simulink model "MATLAB_TEST"  (R2019b)
settings: Solver=FixedStepDiscrete  StartTime=0  StopTime=50  FixedStep=0.0025  RelTol=1e-3
undefined symbols (not defined in the file): BCM_COM_PROC_P20, BCM_COM_PROC_P20_SFW_R2018b, BCM_COM_PROC_P2_5, BCM_COM_PROC_P2_5_SFW_R2018b, BCM_COM_PROC_P5, BCM_COM_PROC_P5_SFW_R2018b, BCMA_ACCU_PT_Conf_Flt, BCMA_ACCU_PT_Unconf_Flt, BCMA_Antiskid_Off_Sanction, BCMA_Avionics_Conf_Flt, BCMA_BCM_CCDL_Conf_Flt, BCMA_BCM_CCDL_Unconf_Flt, BCMA_BCM_DBCU_INHIBITION_Conf_Flt, BCMA_BCM_DBCU_INHIBITION_Unconf_Flt, BCMA_BCP_ALT_Disp_Sw_Conf_Flt, BCMA_BCP_ALT_Disp_Sw_Unconf_Flt, BCMA_BCP_ALT_SW_ON_CMD_Conf_Flt, BCMA_BCP_ALT_SW_ON_CMD_Unconf_Flt, BCMA_BCP_PARK_OFF_SW_CMD_Conf_Flt, BCMA_BCP_PARK_OFF_SW_CMD_Unconf_Flt, BCMA_CF_BSELV_JCL, BCMA_CF_BSELV_JOP, BCMA_CF_BSELV_OC, BCMA_CF_BSELV_SC, BCMA_CF_LH_SV_JCL, BCMA_CF_LH_SV_JOP, BCMA_CF_LH_SV_OC, BCMA_CF_LH_SV_SC, BCMA_CF_PARK_BRK, BCMA_CF_RESIDUAL_PRESS, BCMA_CF_RH_SV_JCL, BCMA_CF_RH_SV_JOP, BCMA_CF_RH_SV_OC, BCMA_CF_RH_SV_SC, BCMA_CF_SELV_JCL, BCMA_CF_SELV_JOP, BCMA_CF_SELV_OC, BCMA_CF_SELV_SC, BCMA_CF_SV_DRIFT, BCMA_DBCU_ALT_MODE_Conf_Flt, BCMA_DBCU_ALT_MODE_Unconf_Flt, BCMA_DBCU_BRK_ORDER_FAIL_Conf_Flt, BCMA_DBCU_BRK_ORDER_FAIL_Unconf_Flt, BCMA_DBCU_Conf_Flt, BCMA_DBCU_DISPATCH_SW_ON_Conf_Flt, BCMA_DBCU_DISPATCH_SW_ON_Unconf_Flt, BCMA_DBCU_FAILED_Conf_Flt, BCMA_DBCU_FAILED_Unconf_Flt, BCMA_DFCS1_Capsule_Validity, BCMA_DFCS1_Label202_Corrupted, BCMA_DFCS1_Label202_Not_Refreshed, BCMA_DFCS1_Label204_Corrupted, BCMA_DFCS1_Label204_Not_Refreshed, BCMA_DFCS1_Label205_Corrupted, BCMA_DFCS1_Label205_Not_Refreshed, BCMA_DFCS1_Label206_Corrupted, BCMA_DFCS1_Label206_Not_Refreshed, BCMA_DFCS1_Label207_Corrupted, BCMA_DFCS1_Label207_Not_Refreshed, BCMA_DFCS3_Capsule_Validity ... (+762)
libraries: simulink x73, lib_MBD_Control x5
(part 8 of 16)

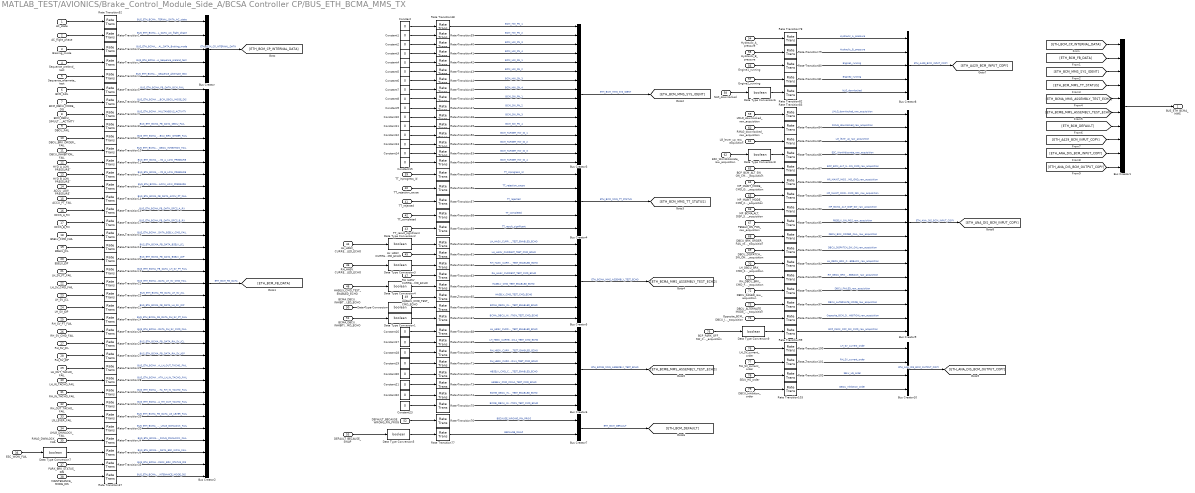
== system MATLAB_TEST/AVIONICS/Brake_Control_Module_Side_A/BCSA Controller CP/BUS_ETH_BCMA_MMS_TX ==
  AC_state : Inport
  AC_flight_phase : Inport  Port=2
  Braking_mode : Inport  Port=3
  Sequence_preland_test : Inport  Port=4
  Sequence_alternate_test : Inport  Port=5
  BCM_FAIL : Inport  Port=6
  BCM_DBCU_MODE_DIS : Inport  Port=7
  BCM_DBCU_SIMULTANEOUS_ACTIVITY : Inport  Port=8
  DBCU_FAIL : Inport  Port=9
  DBCU_BRK_ORDER_FAIL : Inport  Port=10
  DBCU_INHIBITION_FAIL : Inport  Port=11
  HYD_A_LOW_PRESSURE : Inport  Port=12
  HYD_B_LOW_PRESSURE : Inport  Port=13
  ACCU_LOW_PRESSURE : Inport  Port=14
  ACCU_PT_FAIL : Inport  Port=15
  DFCS_A_RX : Inport  Port=16
  DFCS_B_RX : Inport  Port=17
  BSELV_CMD_FAIL : Inport  Port=18
  BSELV_JCL : Inport  Port=19
  BSELV_JOP : Inport  Port=20
  LH_SV_PT_FAIL : Inport  Port=21
  LH_SV_CMD_FAIL : Inport  Port=22
  LH_SV_JCL : Inport  Port=23
  LH_SV_JOP : Inport  Port=24
  RH_SV_PT_FAIL : Inport  Port=25
  RH_SV_CMD_FAIL : Inport  Port=26
  RH_SV_JCL : Inport  Port=27
  RH_SV_JOP : Inport  Port=28
  LH_OUT_TACHO_FAIL : Inport  Port=29
  LH_IN_TACHO_FAIL : Inport  Port=30
  RH_IN_TACHO_FAIL : Inport  Port=31
  RH_OUT_TACHO_FAIL : Inport  Port=32
  LG_LEVER_FAIL : Inport  Port=33
  LMLG_DWNLOCK_FAIL : Inport  Port=34
  RMLG_DWNLOCK_FAIL : Inport  Port=35
  ESC_WOW_FAIL : Inport  Port=36
  PARK_BRK_STATUS_DIS : Inport  Port=37
  MAINTENANCE_MODE_DIS : Inport  Port=38
  TT_inprogress_id : Inport  Port=39
  TT_rejection_cause : Inport  Port=40
  TT_rejected : Inport  Port=41
  TT_completed : Inport  Port=42
  TT_result_significant : Inport  Port=43
  LH_HASV_CURRENT_TEST_ENABLED_ECHO : Inport  Port=44
  LH_HASV_CURRENT_TEST_CMD_ECHO : Inport  Port=45
  RH_HASV_CURRENT_TEST_ENABLED_ECHO : Inport  Port=46
  RH_HASV_CURRENT_TEST_CMD_ECHO : Inport  Port=47
  HASELV_CMD_TEST_ENABLED_ECHO : Inport  Port=48
  HASELV_CMD_TEST_CMD_ECHO : Inport  Port=49
  BCMA_DBCU_INHIBITION_TEST_ENABLED_ECHO : Inport  Port=50
  BCMA_DBCU_INHIBITION_TEST_CMD_ECHO : Inport  Port=51
  DEFAULT_BECAUSE_WRONG_PIN_PROG : Inport  Port=52
  DEFAULT_BECAUSE_SWAP : Inport  Port=53
  Hydraulic_A_pressure : Inport  Port=54
  Hydraulic_B_pressure : Inport  Port=55
  Engine1_running : Inport  Port=56
  Engine2_running : Inport  Port=57
  NLG_downlocked : Inport  Port=58
  LMLG_downlocked_raw_acquisition : Inport  Port=59
  RMLG_downlocked_raw_acquisition : Inport  Port=60
  LG_lever_up_raw_acquisition : Inport  Port=61
  ESC_WonWdiscrete_raw_acquisition : Inport  Port=62
  BCP_BCM_ALT_SW_ON_CMD_raw_acquisition : Inport  Port=63
  MP_MAINT_MODE_CMD_GND_raw_acquisition : Inport  Port=64
  MP_MAINT_MODE_CMD_28V_raw_acquisition : Inport  Port=65
  MP_BCMA_ALT_DISP_SW_raw_acquisition : Inport  Port=66
  PBSELV_ON_POS_raw_acquisition : Inport  Port=67
  DBCU_BRK_ORDER_FAIL_raw_acquisition : Inport  Port=68
  DBCU_DISPATCH_SW_ON_raw_acquisition : Inport  Port=69
  LH_DBCU_BRK_CMD_FEEDBACK_raw_acquisition : Inport  Port=70
  RH_DBCU_BRK_CMD_FEEDBACK_raw_acquisition : Inport  Port=71
  DBCU_FAILED_raw_acquisition : Inport  Port=72
  DBCU_ALTERNATE_MODE_raw_acquisition : Inport  Port=73
  Opposite_BCM_DBCU_INHIBITION_raw_acquisition : Inport  Port=74
  BCP_PARK_OFF_SW_CMD_raw_acquisition : Inport  Port=75
  LH_SV_current_order : Inport  Port=76
  RH_SV_current_order : Inport  Port=77
  SELV_HS_order : Inport  Port=78
  DBCU_Inhibition_order : Inport  Port=79
  Bus Creator : BusCreator  Inputs=5  OutDataTypeStr=Bus: BUS_ETH_BCM_CP_INTERNAL_DATA  NonVirtualBus=on
  Bus Creator1 : BusCreator  Inputs=10  OutDataTypeStr=Bus: BUS_ETH_BCMB_MMS  NonVirtualBus=on
      settings: InheritFromInputs=off
  Bus Creator10 : BusCreator  Inputs=4  OutDataTypeStr=Bus: BUS_ETH_ANA_DIS_BCM_OUTPUT_COPY  NonVirtualBus=on
      settings: InheritFromInputs=off
  Bus Creator2 : BusCreator  Inputs=33  OutDataTypeStr=Bus: BUS_ETH_BCM_FB_DATA  NonVirtualBus=on
      settings: InheritFromInputs=off
  Bus Creator3 : BusCreator  Inputs=16  OutDataTypeStr=Bus: BUS_ETH_BCM_MMS_SYS_IDENT  NonVirtualBus=on
      settings: InheritFromInputs=off
  Bus Creator4 : BusCreator  Inputs=5  OutDataTypeStr=Bus: BUS_ETH_BCM_MMS_TT_STATUS  NonVirtualBus=on
      settings: InheritFromInputs=off
  Bus Creator5 : BusCreator  Inputs=8  OutDataTypeStr=Bus: BUS_ETH_BCMA_MMS_ASSEMBLY_TEST_ECHO  NonVirtualBus=on
      settings: InheritFromInputs=off
  Bus Creator6 : BusCreator  Inputs=8  OutDataTypeStr=Bus: BUS_ETH_BCMB_MMS_ASSEMBLY_TEST_ECHO  NonVirtualBus=on
      settings: InheritFromInputs=off
  Bus Creator7 : BusCreator  Inputs=2  OutDataTypeStr=Bus: BUS_ETH_BCM_DEFAULT  NonVirtualBus=on
      settings: InheritFromInputs=off
  Bus Creator8 : BusCreator  Inputs=5  OutDataTypeStr=Bus: BUS_ETH_A429_BCM_INPUT_COPY  NonVirtualBus=on
      settings: InheritFromInputs=off
  Bus Creator9 : BusCreator  Inputs=17  OutDataTypeStr=Bus: BUS_ETH_ANA_DIS_BCM_INPUT_COPY  NonVirtualBus=on
      settings: InheritFromInputs=off
  Constant{,1..16,18,20,22..23} (21 alike) : Constant  Value=0  OutDataTypeStr=boolean
  Constant17 : Constant  Value=0  OutDataTypeStr=int32
  Constant19 : Constant  Value=0  OutDataTypeStr=int32
  Constant21 : Constant  Value=0  OutDataTypeStr=int32
  Data Type Conversion{,1..9} (10 alike) : DataTypeConversion  OutDataTypeStr=boolean
  Rate Transition{1..103} (103 alike) : RateTransition  Deterministic=off  OutPortSampleTime=1/10
      settings: AttributesFormatString=OutPortSampleTime %<OutPortSampleTime>
  BUS_ETH_BCMA_MMS : Outport  VectorParamsAs1DForOutWhenUnconnected=off
  wires:
  Bus Creator/1 -> [ETH_BCM_CP_INTERNAL_DATA]  "ETH_BCM_CP_INTERNAL_DATA"
  AC_flight_phase/1 -> Rate Transition1/1
  Braking_mode/1 -> Rate Transition2/1
  Sequence_preland_test/1 -> Rate Transition3/1
  Sequence_alternate_test/1 -> Rate Transition4/1
  Bus Creator1/1 -> BUS_ETH_BCMA_MMS/1
  Bus Creator2/1 -> [ETH_BCM_FB_DATA]  "ETH_BCM_FB_DATA"
  BCM_FAIL/1 -> Rate Transition5/1
  BCM_DBCU_MODE_DIS/1 -> Rate Transition6/1
  BCM_DBCU_SIMULTANEOUS_ACTIVITY/1 -> Rate Transition7/1
  DBCU_FAIL/1 -> Rate Transition8/1
  DBCU_BRK_ORDER_FAIL/1 -> Rate Transition9/1
  DBCU_INHIBITION_FAIL/1 -> Rate Transition10/1
  HYD_A_LOW_PRESSURE/1 -> Rate Transition11/1
  HYD_B_LOW_PRESSURE/1 -> Rate Transition12/1
  ACCU_LOW_PRESSURE/1 -> Rate Transition13/1
  ACCU_PT_FAIL/1 -> Rate Transition14/1
  DFCS_A_RX/1 -> Rate Transition15/1
  DFCS_B_RX/1 -> Rate Transition17/1
  BSELV_CMD_FAIL/1 -> Rate Transition16/1
  BSELV_JCL/1 -> Rate Transition18/1
  BSELV_JOP/1 -> Rate Transition20/1
  LH_SV_PT_FAIL/1 -> Rate Transition19/1
  LH_SV_CMD_FAIL/1 -> Rate Transition21/1
  LH_SV_JCL/1 -> Rate Transition23/1
  LH_SV_JOP/1 -> Rate Transition22/1
  RH_SV_PT_FAIL/1 -> Rate Transition24/1
  RH_SV_CMD_FAIL/1 -> Rate Transition26/1
  RH_SV_JCL/1 -> Rate Transition25/1
  RH_SV_JOP/1 -> Rate Transition27/1
  LH_OUT_TACHO_FAIL/1 -> Rate Transition29/1
  LH_IN_TACHO_FAIL/1 -> Rate Transition28/1
  RH_IN_TACHO_FAIL/1 -> Rate Transition30/1
  RH_OUT_TACHO_FAIL/1 -> Rate Transition31/1
  LG_LEVER_FAIL/1 -> Rate Transition33/1
  LMLG_DWNLOCK_FAIL/1 -> Rate Transition32/1
  RMLG_DWNLOCK_FAIL/1 -> Rate Transition34/1
  ESC_WOW_FAIL/1 -> Data Type Conversion7/1
  PARK_BRK_STATUS_DIS/1 -> Rate Transition35/1
  MAINTENANCE_MODE_DIS/1 -> Rate Transition37/1
  Constant/1 -> Rate Transition38/1
  Constant1/1 -> Rate Transition39/1
  Constant2/1 -> Rate Transition40/1
  Constant3/1 -> Rate Transition41/1
  Constant4/1 -> Rate Transition42/1
  Constant5/1 -> Rate Transition43/1
  Constant6/1 -> Rate Transition44/1
  Constant7/1 -> Rate Transition45/1
  Constant8/1 -> Rate Transition46/1
  Constant9/1 -> Rate Transition47/1
  Constant10/1 -> Rate Transition48/1
  Constant11/1 -> Rate Transition49/1
  Constant12/1 -> Rate Transition50/1
  Constant13/1 -> Rate Transition51/1
  Constant14/1 -> Rate Transition53/1
  Constant15/1 -> Rate Transition54/1
  [ETH_BCM_CP_INTERNAL_DATA] -> Bus Creator1/1
  [ETH_BCM_FB_DATA] -> Bus Creator1/2
  Bus Creator3/1 -> [ETH_BCM_MMS_SYS_IDENT]  "ETH_BCM_MMS_SYS_IDENT"
  [ETH_BCM_MMS_SYS_IDENT] -> Bus Creator1/3
  TT_result_significant/1 -> Rate Transition59/1
  TT_completed/1 -> Rate Transition58/1
  TT_rejected/1 -> Rate Transition57/1
  TT_rejection_cause/1 -> Rate Transition56/1
  TT_inprogress_id/1 -> Rate Transition55/1
  Bus Creator4/1 -> [ETH_BCM_MMS_TT_STATUS]  "ETH_BCM_MMS_TT_STATUS"
  [ETH_BCM_MMS_TT_STATUS] -> Bus Creator1/4
  Bus Creator5/1 -> [ETH_BCMA_MMS_ASSEMBLY_TEST_ECHO]  "ETH_BCMA_MMS_ASSEMBLY_TEST_ECHO"
  [ETH_BCMA_MMS_ASSEMBLY_TEST_ECHO] -> Bus Creator1/5
  LH_HASV_CURRENT_TEST_ENABLED_ECHO/1 -> Data Type Conversion2/1
  LH_HASV_CURRENT_TEST_CMD_ECHO/1 -> Rate Transition61/1
  RH_HASV_CURRENT_TEST_ENABLED_ECHO/1 -> Data Type Conversion3/1
  RH_HASV_CURRENT_TEST_CMD_ECHO/1 -> Rate Transition63/1
  HASELV_CMD_TEST_ENABLED_ECHO/1 -> Data Type Conversion4/1
  HASELV_CMD_TEST_CMD_ECHO/1 -> Rate Transition65/1
  BCMA_DBCU_INHIBITION_TEST_ENABLED_ECHO/1 -> Data Type Conversion/1
  BCMA_DBCU_INHIBITION_TEST_CMD_ECHO/1 -> Data Type Conversion1/1
  Constant23/1 -> Rate Transition75/1
  Constant22/1 -> Rate Transition74/1
  Constant21/1 -> Rate Transition73/1
  Constant20/1 -> Rate Transition72/1
  Constant19/1 -> Rate Transition71/1
  Constant18/1 -> Rate Transition70/1
  Constant17/1 -> Rate Transition69/1
  Constant16/1 -> Rate Transition68/1
  Bus Creator6/1 -> [ETH_BCMB_MMS_ASSEMBLY_TEST_ECHO]  "ETH_BCMB_MMS_ASSEMBLY_TEST_ECHO"
  [ETH_BCMB_MMS_ASSEMBLY_TEST_ECHO] -> Bus Creator1/6
  DEFAULT_BECAUSE_SWAP/1 -> Data Type Conversion5/1
  DEFAULT_BECAUSE_WRONG_PIN_PROG/1 -> Rate Transition76/1
  Bus Creator7/1 -> [ETH_BCM_DEFAULT]  "ETH_BCM_DEFAULT"
  [ETH_BCM_DEFAULT] -> Bus Creator1/7
  Rate Transition52/1 -> Bus Creator/1  "BUS_ETH_BCMA_CP_INTERNAL_DATA_AC_state"
  Rate Transition1/1 -> Bus Creator/2  "BUS_ETH_BCMA_CP_INTERNAL_DATA_AC_flight_phase"
  Rate Transition2/1 -> Bus Creator/3  "BUS_ETH_BCMA_CP_INTERNAL_DATA_Braking_mode"
  Rate Transition3/1 -> Bus Creator/4  "BUS_ETH_BCMA_CP_INTERNAL_DATA_Sequence_preland_test"
  Rate Transition4/1 -> Bus Creator/5  "BUS_ETH_BCMA_CP_INTERNAL_DATA_Sequence_alternate_test"
  Rate Transition5/1 -> Bus Creator2/1  "BUS_ETH_BCMA_FB_DATA_BCM_FAIL"
  Rate Transition6/1 -> Bus Creator2/2  "BUS_ETH_BCMA_FB_DATA_BCM_DBCU_MODE_DIS"
  Rate Transition7/1 -> Bus Creator2/3  "BUS_ETH_BCMA_FB_DATA_BCM_DBCU_SIMULTANEOUS_ACTIVITY"
  Rate Transition8/1 -> Bus Creator2/4  "BUS_ETH_BCMA_FB_DATA_DBCU_FAIL"
  Rate Transition9/1 -> Bus Creator2/5  "BUS_ETH_BCMA_FB_DATA_DBCU_BRK_ORDER_FAIL"
  Rate Transition10/1 -> Bus Creator2/6  "BUS_ETH_BCMA_FB_DATA_DBCU_INHIBITION_FAIL"
  Rate Transition11/1 -> Bus Creator2/7  "BUS_ETH_BCMA_FB_DATA_HYD_A_LOW_PRESSURE"
  Rate Transition12/1 -> Bus Creator2/8  "BUS_ETH_BCMA_FB_DATA_HYD_B_LOW_PRESSURE"
  Rate Transition13/1 -> Bus Creator2/9  "BUS_ETH_BCMA_FB_DATA_ACCU_LOW_PRESSURE"
  Rate Transition14/1 -> Bus Creator2/10  "BUS_ETH_BCMA_FB_DATA_ACCU_PT_FAIL"
  Rate Transition16/1 -> Bus Creator2/13  "BUS_ETH_BCMA_FB_DATA_BSELV_CMD_FAIL"
  Rate Transition15/1 -> Bus Creator2/11  "BUS_ETH_BCMA_FB_DATA_DFCS_A_RX"
  Rate Transition17/1 -> Bus Creator2/12  "BUS_ETH_BCMA_FB_DATA_DFCS_B_RX"
  Rate Transition18/1 -> Bus Creator2/14  "BUS_ETH_BCMA_FB_DATA_BSELV_JCL"
  Rate Transition20/1 -> Bus Creator2/15  "BUS_ETH_BCMA_FB_DATA_BSELV_JOP"
  Rate Transition19/1 -> Bus Creator2/16  "BUS_ETH_BCMA_FB_DATA_LH_SV_PT_FAIL"
  Rate Transition23/1 -> Bus Creator2/18  "BUS_ETH_BCMA_FB_DATA_LH_SV_JCL"
  Rate Transition22/1 -> Bus Creator2/19  "BUS_ETH_BCMA_FB_DATA_LH_SV_JOP"
  Rate Transition21/1 -> Bus Creator2/17  "BUS_ETH_BCMA_FB_DATA_LH_SV_CMD_FAIL"
  Rate Transition26/1 -> Bus Creator2/21  "BUS_ETH_BCMA_FB_DATA_RH_SV_CMD_FAIL"
  Rate Transition25/1 -> Bus Creator2/22  "BUS_ETH_BCMA_FB_DATA_RH_SV_JCL"
  Rate Transition24/1 -> Bus Creator2/20  "BUS_ETH_BCMA_FB_DATA_RH_SV_PT_FAIL"
  Rate Transition29/1 -> Bus Creator2/24  "BUS_ETH_BCMA_FB_DATA_LH_OUT_TACHO_FAIL"
  Rate Transition27/1 -> Bus Creator2/23  "BUS_ETH_BCMA_FB_DATA_RH_SV_JOP"
  Rate Transition28/1 -> Bus Creator2/25  "BUS_ETH_BCMA_FB_DATA_LH_IN_TACHO_FAIL"
  Rate Transition36/1 -> Bus Creator2/31  "BUS_ETH_BCMA_FB_DATA_ESC_WOW_FAIL"
  Rate Transition35/1 -> Bus Creator2/32  "BUS_ETH_BCMA_FB_DATA_PARK_BRK_STATUS_DIS"
  Rate Transition34/1 -> Bus Creator2/30  "BUS_ETH_BCMA_FB_DATA_RMLG_DWNLOCK_FAIL"
  Rate Transition31/1 -> Bus Creator2/27  "BUS_ETH_BCMA_FB_DATA_RH_OUT_TACHO_FAIL"
  Rate Transition32/1 -> Bus Creator2/29  "BUS_ETH_BCMA_FB_DATA_LMLG_DWNLOCK_FAIL"
  Rate Transition30/1 -> Bus Creator2/26  "BUS_ETH_BCMA_FB_DATA_RH_IN_TACHO_FAIL"
  Rate Transition33/1 -> Bus Creator2/28  "BUS_ETH_BCMA_FB_DATA_LG_LEVER_FAIL"
  Rate Transition37/1 -> Bus Creator2/33  "BUS_ETH_BCMA_FB_DATA_MAINTENANCE_MODE_DIS"
  AC_state/1 -> Rate Transition52/1
  Rate Transition38/1 -> Bus Creator3/1  "BCM_HW_PN_1"
  Rate Transition39/1 -> Bus Creator3/2  "BCM_HW_PN_2"
  Rate Transition40/1 -> Bus Creator3/3  "BCM_HW_PN_3"
  Rate Transition41/1 -> Bus Creator3/4  "BCM_HW_PN_4"
  Rate Transition42/1 -> Bus Creator3/5  "BCM_HW_SN_1"
  Rate Transition43/1 -> Bus Creator3/6  "BCM_HW_SN_2"
  Rate Transition44/1 -> Bus Creator3/7  "BCM_HW_SN_3"
  Rate Transition45/1 -> Bus Creator3/8  "BCM_HW_SN_4"
  Rate Transition46/1 -> Bus Creator3/9  "BCM_SW_PN_1"
  Rate Transition47/1 -> Bus Creator3/10  "BCM_SW_PN_2"
  Rate Transition50/1 -> Bus Creator3/13  "BCM_TARGET_HW_ID_1"
  Rate Transition49/1 -> Bus Creator3/12  "BCM_SW_PN_4"
  Rate Transition48/1 -> Bus Creator3/11  "BCM_SW_PN_3"
  Rate Transition51/1 -> Bus Creator3/14  "BCM_TARGET_HW_ID_2"
  Rate Transition53/1 -> Bus Creator3/15  "BCM_TARGET_HW_ID_3"
  Rate Transition54/1 -> Bus Creator3/16  "BCM_TARGET_HW_ID_4"
  Rate Transition55/1 -> Bus Creator4/1  "TT_inprogress_id"
  Rate Transition56/1 -> Bus Creator4/2  "TT_rejection_cause"
  Rate Transition57/1 -> Bus Creator4/3  "TT_rejected"
  Rate Transition58/1 -> Bus Creator4/4  "TT_completed"
  Rate Transition59/1 -> Bus Creator4/5  "TT_result_significant"
  Rate Transition60/1 -> Bus Creator5/1  "LH_HASV_CURRENT_TEST_ENABLED_ECHO"
  Rate Transition61/1 -> Bus Creator5/2  "LH_HASV_CURRENT_TEST_CMD_ECHO"
  Rate Transition62/1 -> Bus Creator5/3  "RH_HASV_CURRENT_TEST_ENABLED_ECHO"
  Rate Transition63/1 -> Bus Creator5/4  "RH_HASV_CURRENT_TEST_CMD_ECHO"
  Rate Transition64/1 -> Bus Creator5/5  "HASELV_CMD_TEST_ENABLED_ECHO"
  Rate Transition65/1 -> Bus Creator5/6  "HASELV_CMD_TEST_CMD_ECHO"
  Rate Transition66/1 -> Bus Creator5/7  "BCMA_DBCU_INHIBITION_TEST_ENABLED_ECHO"
  Rate Transition67/1 -> Bus Creator5/8  "BCMA_DBCU_INHIBITION_TEST_CMD_ECHO"
  Rate Transition68/1 -> Bus Creator6/1  "LH_HBSV_CURRENT_COIL1_TEST_ENABLED_ECHO"
  Rate Transition69/1 -> Bus Creator6/2  "LH_HBSV_CURRENT_COIL1_TEST_CMD_ECHO"
  Rate Transition70/1 -> Bus Creator6/3  "RH_HBSV_CURRENT_COIL1_TEST_ENABLED_ECHO"
  Rate Transition71/1 -> Bus Creator6/4  "RH_HBSV_CURRENT_COIL1_TEST_CMD_ECHO"
  Rate Transition72/1 -> Bus Creator6/5  "HBSELV_CMD_COIL1_TEST_ENABLED_ECHO"
  Rate Transition73/1 -> Bus Creator6/6  "HBSELV_CMD_COIL1_TEST_CMD_ECHO"
  Rate Transition74/1 -> Bus Creator6/7  "BCMB_DBCU_INHIBITION_TEST_ENABLED_ECHO"
  Rate Transition75/1 -> Bus Creator6/8  "BCMB_DBCU_INHIBITION_TEST_CMD_ECHO"
  Rate Transition76/1 -> Bus Creator7/1  "BECAUSE_WRONG_PIN_PROG"
  Rate Transition77/1 -> Bus Creator7/2  "BECAUSE_SWAP"
  Hydraulic_A_pressure/1 -> Rate Transition78/1
  Hydraulic_B_pressure/1 -> Rate Transition79/1
  Engine1_running/1 -> Rate Transition80/1
  Engine2_running/1 -> Rate Transition81/1
  NLG_downlocked/1 -> Data Type Conversion6/1
  Rate Transition78/1 -> Bus Creator8/1  "Hydraulic_A_pressure"
  Rate Transition79/1 -> Bus Creator8/2  "Hydraulic_B_pressure"
  Rate Transition80/1 -> Bus Creator8/3  "Engine1_running"
  Rate Transition81/1 -> Bus Creator8/4  "Engine2_running"
  Rate Transition82/1 -> Bus Creator8/5  "NLG_downlocked"
  Bus Creator8/1 -> [ETH_A429_BCM_INPUT_COPY]  "ETH_A429_BCM_INPUT_COPY"
  [ETH_A429_BCM_INPUT_COPY] -> Bus Creator1/8
  Rate Transition83/1 -> Bus Creator9/1  "LMLG_downlocked_raw_acquisition"
  Rate Transition84/1 -> Bus Creator9/2  "RMLG_downlocked_raw_acquisition"
  Rate Transition86/1 -> Bus Creator9/4  "ESC_WonWdiscrete_raw_acquisition"
  Rate Transition85/1 -> Bus Creator9/3  "LG_lever_up_raw_acquisition"
  Rate Transition87/1 -> Bus Creator9/5  "BCP_BCM_ALT_SW_ON_CMD_raw_acquisition"
  Rate Transition88/1 -> Bus Creator9/6  "MP_MAINT_MODE_CMD_GND_raw_acquisition"
  Rate Transition89/1 -> Bus Creator9/7  "MP_MAINT_MODE_CMD_28V_raw_acquisition"
  Rate Transition90/1 -> Bus Creator9/8  "MP_BCMA_ALT_DISP_SW_raw_acquisition"
  Rate Transition91/1 -> Bus Creator9/9  "PBSELV_ON_POS_raw_acquisition"
  Rate Transition92/1 -> Bus Creator9/10  "DBCU_BRK_ORDER_FAIL_raw_acquisition"
  Rate Transition93/1 -> Bus Creator9/11  "DBCU_DISPATCH_SW_ON_raw_acquisition"
  Rate Transition94/1 -> Bus Creator9/12  "LH_DBCU_BRK_CMD_FEEDBACK_raw_acquisition"
  Rate Transition95/1 -> Bus Creator9/13  "RH_DBCU_BRK_CMD_FEEDBACK_raw_acquisition"
  Rate Transition96/1 -> Bus Creator9/14  "DBCU_FAILED_raw_acquisition"
  Rate Transition97/1 -> Bus Creator9/15  "DBCU_ALTERNATE_MODE_raw_acquisition"
  Rate Transition98/1 -> Bus Creator9/16  "Opposite_BCM_DBCU_INHIBITION_raw_acquisition"
  Rate Transition99/1 -> Bus Creator9/17  "BCP_PARK_OFF_SW_CMD_raw_acquisition"
  LMLG_downlocked_raw_acquisition/1 -> Rate Transition83/1
  RMLG_downlocked_raw_acquisition/1 -> Rate Transition84/1
  LG_lever_up_raw_acquisition/1 -> Rate Transition85/1
  ESC_WonWdiscrete_raw_acquisition/1 -> Data Type Conversion8/1
  MP_MAINT_MODE_CMD_GND_raw_acquisition/1 -> Rate Transition88/1
  BCP_BCM_ALT_SW_ON_CMD_raw_acquisition/1 -> Rate Transition87/1
  MP_MAINT_MODE_CMD_28V_raw_acquisition/1 -> Rate Transition89/1
  MP_BCMA_ALT_DISP_SW_raw_acquisition/1 -> Rate Transition90/1
  PBSELV_ON_POS_raw_acquisition/1 -> Rate Transition91/1
  DBCU_BRK_ORDER_FAIL_raw_acquisition/1 -> Rate Transition92/1
  DBCU_DISPATCH_SW_ON_raw_acquisition/1 -> Rate Transition93/1
  LH_DBCU_BRK_CMD_FEEDBACK_raw_acquisition/1 -> Rate Transition94/1
  RH_DBCU_BRK_CMD_FEEDBACK_raw_acquisition/1 -> Rate Transition95/1
  DBCU_FAILED_raw_acquisition/1 -> Rate Transition96/1
  DBCU_ALTERNATE_MODE_raw_acquisition/1 -> Rate Transition97/1
  Opposite_BCM_DBCU_INHIBITION_raw_acquisition/1 -> Rate Transition98/1
  BCP_PARK_OFF_SW_CMD_raw_acquisition/1 -> Data Type Conversion9/1
  Bus Creator9/1 -> [ETH_ANA_DIS_BCM_INPUT_COPY]  "ETH_ANA_DIS_BCM_INPUT_COPY"
  [ETH_ANA_DIS_BCM_INPUT_COPY] -> Bus Creator1/9
  Bus Creator10/1 -> [ETH_ANA_DIS_BCM_OUTPUT_COPY]  "ETH_ANA_DIS_BCM_OUTPUT_COPY"
  [ETH_ANA_DIS_BCM_OUTPUT_COPY] -> Bus Creator1/10
  Rate Transition100/1 -> Bus Creator10/1  "LH_SV_current_order"
  LH_SV_current_order/1 -> Rate Transition100/1
  RH_SV_current_order/1 -> Rate Transition101/1
  SELV_HS_order/1 -> Rate Transition102/1
  DBCU_Inhibition_order/1 -> Rate Transition103/1
  Rate Transition101/1 -> Bus Creator10/2  "RH_SV_current_order"
  Rate Transition102/1 -> Bus Creator10/3  "SELV_HS_order"
  Rate Transition103/1 -> Bus Creator10/4  "DBCU_Inhibition_order"
  Data Type Conversion/1 -> Rate Transition66/1
  Data Type Conversion1/1 -> Rate Transition67/1
  Data Type Conversion2/1 -> Rate Transition60/1
  Data Type Conversion3/1 -> Rate Transition62/1
  Data Type Conversion4/1 -> Rate Transition64/1
  Data Type Conversion5/1 -> Rate Transition77/1
  Data Type Conversion6/1 -> Rate Transition82/1
  Data Type Conversion7/1 -> Rate Transition36/1
  Data Type Conversion8/1 -> Rate Transition86/1
  Data Type Conversion9/1 -> Rate Transition99/1

== system MATLAB_TEST/AVIONICS/Brake_Control_Module_Side_A/BCSA Controller CP/COM_CAN_MON_TX ==
  V_BCM_COM_Braking_Norm_FT_Seq : Inport  SampleTime=0.005
  V_BCM_COM_Braking_Alt_FT_Seq : Inport  Port=2  SampleTime=0.005
  V_BCM_COM_BCM_Validity : Inport  Port=3  SampleTime=0.005
  V_BCM_COM_Norm_Brkg_Availability : Inport  Port=4  SampleTime=0.005
  Bus Creator : BusCreator  Inputs=4
  COM_CAN_MON : Outport  OutputWhenDisabled=reset  InitialOutput=0  VectorParamsAs1DForOutWhenUnconnected=off
      settings: AttributesFormatString=|
      | OutputWhenDisabled %<OutputWhenDisabled>
      | InitialOutput %<InitialOutput>
  wires:
  V_BCM_COM_Braking_Norm_FT_Seq/1 -> Bus Creator/1
  V_BCM_COM_Braking_Alt_FT_Seq/1 -> Bus Creator/2
  V_BCM_COM_BCM_Validity/1 -> Bus Creator/3
  V_BCM_COM_Norm_Brkg_Availability/1 -> Bus Creator/4
  Bus Creator/1 -> COM_CAN_MON/1

== system MATLAB_TEST/AVIONICS/Brake_Control_Module_Side_A/BCSA Controller CP/DBCU Inhibition Failure Mode ==
  DBCU_Inhib_Order : Inport
  Erroneous_DBCU_Activation_Off : Inport  Port=2  SampleTime=0.02
  Erroneous_DBCU_Activation_On : Inport  Port=3  SampleTime=0.02
  AIG3 : lib_MBD_Control/Logics/Signal Routing/AIG3  Tag=AIG4
      settings: SourceProductName=MBD
  Constant1 : Constant  Value=0  OutDataTypeStr=boolean  SampleTime=0.02
  Constant58 : Constant  OutDataTypeStr=boolean  SampleTime=0.02
  DBCU_INHIBITION : Outport  VectorParamsAs1DForOutWhenUnconnected=off
  wires:
  DBCU_Inhib_Order/1 -> AIG3/5
  Erroneous_DBCU_Activation_Off/1 -> AIG3/1
  Erroneous_DBCU_Activation_On/1 -> AIG3/2
  AIG3/1 -> DBCU_INHIBITION/1
  Constant58/1 -> AIG3/3
  Constant1/1 -> AIG3/4

== system MATLAB_TEST/AVIONICS/Brake_Control_Module_Side_A/BCSA Controller CP/DFCS1_Label204_Validity ==
  Capsule_Validity : Inport
  Label204_Not_Refreshed : Inport  Port=2
  Label204_Corrupted : Inport  Port=3
  Label204_SSM : Inport  Port=4
  Compare To Constant : simulink/Logic and Bit Operations/Compare To Constant  relop=~=  const=0  OutDataTypeStr=boolean
  Compare To Zero : simulink/Logic and Bit Operations/Compare To Zero  relop===  OutDataTypeStr=boolean
  Logical Operator : Logic  Operator=OR  Inputs=4  AllPortsSameDT=off  OutDataTypeStr=boolean
  Logical Operator5 : Logic  Operator=NOT  AllPortsSameDT=off  OutDataTypeStr=boolean
  Mux{16,18,20,22} (4 alike) : Mux  Inputs=3
  WOWs_Val_Val : Outport  VectorParamsAs1DForOutWhenUnconnected=off
  LMLG_WOWs_Val : Outport  Port=2  VectorParamsAs1DForOutWhenUnconnected=off
  RMLG_WOWs_Val : Outport  Port=3  VectorParamsAs1DForOutWhenUnconnected=off
  NLG_WOWs_Val : Outport  Port=4  VectorParamsAs1DForOutWhenUnconnected=off
  TLA_Above_Idle_Val : Outport  Port=5  VectorParamsAs1DForOutWhenUnconnected=off
  DCL_Inhibition_Val : Outport  Port=6  VectorParamsAs1DForOutWhenUnconnected=off
  ALT_Mode_1_Val : Outport  Port=7  VectorParamsAs1DForOutWhenUnconnected=off
  ALT_Mode_2_Val : Outport  Port=8  VectorParamsAs1DForOutWhenUnconnected=off
  wires:
  Logical Operator/1 -> Logical Operator5/1
  Mux16/1 -> WOWs_Val_Val/1
  Mux18/1 -> LMLG_WOWs_Val/1
  Mux20/1 -> RMLG_WOWs_Val/1
  Mux22/1 -> NLG_WOWs_Val/1
  Capsule_Validity/1 -> Compare To Zero/1
  Compare To Zero/1 -> Logical Operator/1
  Label204_Not_Refreshed/1 -> Logical Operator/2
  Label204_SSM/1 -> Compare To Constant/1
  Label204_Corrupted/1 -> Logical Operator/3
  Logical Operator5/1 -> ALT_Mode_2_Val/1, ALT_Mode_1_Val/1, DCL_Inhibition_Val/1, TLA_Above_Idle_Val/1, Mux22/3, Mux22/2, Mux22/1, Mux20/3, Mux20/2, Mux20/1, Mux18/3, Mux18/2, Mux18/1, Mux16/3, Mux16/2, Mux16/1
  Compare To Constant/1 -> Logical Operator/4

== system MATLAB_TEST/AVIONICS/Brake_Control_Module_Side_A/BCSA Controller CP/DFCS1_Label205_Validity ==
  Capsule_Validity : Inport
  Label205_Not_Refreshed : Inport  Port=2
  Label205_Corrupted : Inport  Port=3
  Label205_SSM : Inport  Port=4
  DFCSA_Long_Accel : Inport  Port=5
  Compare To Constant : simulink/Logic and Bit Operations/Compare To Constant  relop=~=  const=3.0  OutDataTypeStr=boolean
  Compare To Constant3 : simulink/Logic and Bit Operations/Compare To Constant  relop=<  const=-4  OutDataTypeStr=boolean
  Compare To Constant4 : simulink/Logic and Bit Operations/Compare To Constant  relop=>  const=4  OutDataTypeStr=boolean
  Compare To Zero : simulink/Logic and Bit Operations/Compare To Zero  relop===  OutDataTypeStr=boolean
  Logical Operator1 : Logic  Operator=OR  Inputs=6  AllPortsSameDT=off  OutDataTypeStr=boolean
  Logical Operator5 : Logic  Operator=NOT  AllPortsSameDT=off  OutDataTypeStr=boolean
  Long_Accel_Val : Outport  VectorParamsAs1DForOutWhenUnconnected=off
  wires:
  Capsule_Validity/1 -> Compare To Zero/1
  Compare To Zero/1 -> Logical Operator1/1
  Label205_Not_Refreshed/1 -> Logical Operator1/2
  Logical Operator1/1 -> Logical Operator5/1
  Label205_SSM/1 -> Compare To Constant/1
  Label205_Corrupted/1 -> Logical Operator1/3
  Compare To Constant/1 -> Logical Operator1/4
  Compare To Constant3/1 -> Logical Operator1/5
  DFCSA_Long_Accel/1 -> Compare To Constant4/1, Compare To Constant3/1
  Compare To Constant4/1 -> Logical Operator1/6
  Logical Operator5/1 -> Long_Accel_Val/1

== system MATLAB_TEST/AVIONICS/Brake_Control_Module_Side_A/BCSA Controller CP/DFCS1_Label206_Validity ==
  Capsule_Validity : Inport
  Label206_Not_Refreshed : Inport  Port=2
  Label206_Corrupted : Inport  Port=3
  Label206_SSM : Inport  Port=4
  DFCSA_Gnd_Spd : Inport  Port=5
  Compare To Constant : simulink/Logic and Bit Operations/Compare To Constant  relop=~=  const=3.0  OutDataTypeStr=boolean
  Compare To Constant3 : simulink/Logic and Bit Operations/Compare To Constant  relop=<  const=0  OutDataTypeStr=boolean
  Compare To Constant4 : simulink/Logic and Bit Operations/Compare To Constant  relop=>  const=4096  OutDataTypeStr=boolean
  Compare To Zero : simulink/Logic and Bit Operations/Compare To Zero  relop===  OutDataTypeStr=boolean
  Logical Operator : Logic  Operator=OR  Inputs=6  AllPortsSameDT=off  OutDataTypeStr=boolean
  Logical Operator5 : Logic  Operator=NOT  AllPortsSameDT=off  OutDataTypeStr=boolean
  Gnd_Spd_Val : Outport  VectorParamsAs1DForOutWhenUnconnected=off
  wires:
  Logical Operator/1 -> Logical Operator5/1
  Label206_Not_Refreshed/1 -> Logical Operator/2
  Compare To Zero/1 -> Logical Operator/1
  Capsule_Validity/1 -> Compare To Zero/1
  Label206_SSM/1 -> Compare To Constant/1
  Label206_Corrupted/1 -> Logical Operator/3
  Compare To Constant/1 -> Logical Operator/4
  Compare To Constant3/1 -> Logical Operator/5
  Compare To Constant4/1 -> Logical Operator/6
  DFCSA_Gnd_Spd/1 -> Compare To Constant4/1, Compare To Constant3/1
  Logical Operator5/1 -> Gnd_Spd_Val/1

== system MATLAB_TEST/AVIONICS/Brake_Control_Module_Side_A/BCSA Controller CP/DFCS1_Label207_Validity ==
  Capsule_Validity : Inport
  Label207_Not_Refreshed : Inport  Port=2
  Label207_Corrupted : Inport  Port=3
  Label207_SSM : Inport  Port=4
  DFCSA_Pitch_Ang : Inport  Port=5
  Compare To Constant : simulink/Logic and Bit Operations/Compare To Constant  relop=~=  const=3.0  OutDataTypeStr=boolean
  Compare To Constant3 : simulink/Logic and Bit Operations/Compare To Constant  relop=<  const=-90  OutDataTypeStr=boolean
  Compare To Constant4 : simulink/Logic and Bit Operations/Compare To Constant  relop=>  const=90  OutDataTypeStr=boolean
  Compare To Zero : simulink/Logic and Bit Operations/Compare To Zero  relop===  OutDataTypeStr=boolean
  Logical Operator1 : Logic  Operator=OR  Inputs=6  AllPortsSameDT=off  OutDataTypeStr=boolean
  Logical Operator5 : Logic  Operator=NOT  AllPortsSameDT=off  OutDataTypeStr=boolean
  Pitch_Ang_Val : Outport  VectorParamsAs1DForOutWhenUnconnected=off
  wires:
  Capsule_Validity/1 -> Compare To Zero/1
  Compare To Zero/1 -> Logical Operator1/1
  Label207_Not_Refreshed/1 -> Logical Operator1/2
  Logical Operator1/1 -> Logical Operator5/1
  Label207_SSM/1 -> Compare To Constant/1
  Label207_Corrupted/1 -> Logical Operator1/3
  Compare To Constant/1 -> Logical Operator1/4
  Compare To Constant3/1 -> Logical Operator1/5
  DFCSA_Pitch_Ang/1 -> Compare To Constant4/1, Compare To Constant3/1
  Compare To Constant4/1 -> Logical Operator1/6
  Logical Operator5/1 -> Pitch_Ang_Val/1

== system MATLAB_TEST/AVIONICS/Brake_Control_Module_Side_A/BCSA Controller CP/DFCS3_Label204_Validity ==
  Capsule_Validity : Inport
  Label204_Not_Refreshed : Inport  Port=2
  Label204_Corrupted : Inport  Port=3
  Label204_SSM : Inport  Port=4
  Compare To Constant : simulink/Logic and Bit Operations/Compare To Constant  relop=~=  const=0  OutDataTypeStr=boolean
  Compare To Zero : simulink/Logic and Bit Operations/Compare To Zero  relop===  OutDataTypeStr=boolean
  Logical Operator : Logic  Operator=OR  Inputs=4  AllPortsSameDT=off  OutDataTypeStr=boolean
  Logical Operator5 : Logic  Operator=NOT  AllPortsSameDT=off  OutDataTypeStr=boolean
  Mux{16,18,20,22} (4 alike) : Mux  Inputs=3
  WOWs_Val_Val : Outport  VectorParamsAs1DForOutWhenUnconnected=off
  LMLG_WOWs_Val : Outport  Port=2  VectorParamsAs1DForOutWhenUnconnected=off
  RMLG_WOWs_Val : Outport  Port=3  VectorParamsAs1DForOutWhenUnconnected=off
  NLG_WOWs_Val : Outport  Port=4  VectorParamsAs1DForOutWhenUnconnected=off
  TLA_Above_Idle_Val : Outport  Port=5  VectorParamsAs1DForOutWhenUnconnected=off
  DCL_Inhibition_Val : Outport  Port=6  VectorParamsAs1DForOutWhenUnconnected=off
  ALT_Mode_1_Val : Outport  Port=7  VectorParamsAs1DForOutWhenUnconnected=off
  ALT_Mode_2_Val : Outport  Port=8  VectorParamsAs1DForOutWhenUnconnected=off
  wires:
  Label204_Corrupted/1 -> Logical Operator/3
  Mux22/1 -> NLG_WOWs_Val/1
  Logical Operator/1 -> Logical Operator5/1
  Label204_Not_Refreshed/1 -> Logical Operator/2
  Mux20/1 -> RMLG_WOWs_Val/1
  Capsule_Validity/1 -> Compare To Zero/1
  Label204_SSM/1 -> Compare To Constant/1
  Mux16/1 -> WOWs_Val_Val/1
  Mux18/1 -> LMLG_WOWs_Val/1
  Compare To Zero/1 -> Logical Operator/1
  Logical Operator5/1 -> ALT_Mode_2_Val/1, ALT_Mode_1_Val/1, DCL_Inhibition_Val/1, TLA_Above_Idle_Val/1, Mux22/3, Mux22/2, Mux22/1, Mux20/3, Mux20/2, Mux20/1, Mux18/3, Mux18/2, Mux18/1, Mux16/3, Mux16/2, Mux16/1
  Compare To Constant/1 -> Logical Operator/4

== system MATLAB_TEST/AVIONICS/Brake_Control_Module_Side_A/BCSA Controller CP/DFCS3_Label205_Validity ==
  Capsule_Validity : Inport
  Label205_Not_Refreshed : Inport  Port=2
  Label205_Corrupted : Inport  Port=3
  Label205_SSM : Inport  Port=4
  DFCSB_Long_Accel : Inport  Port=5
  Compare To Constant : simulink/Logic and Bit Operations/Compare To Constant  relop=~=  const=3.0  OutDataTypeStr=boolean
  Compare To Constant3 : simulink/Logic and Bit Operations/Compare To Constant  relop=<  const=-4  OutDataTypeStr=boolean
  Compare To Constant4 : simulink/Logic and Bit Operations/Compare To Constant  relop=>  const=4  OutDataTypeStr=boolean
  Compare To Zero : simulink/Logic and Bit Operations/Compare To Zero  relop===  OutDataTypeStr=boolean
  Logical Operator1 : Logic  Operator=OR  Inputs=6  AllPortsSameDT=off  OutDataTypeStr=boolean
  Logical Operator5 : Logic  Operator=NOT  AllPortsSameDT=off  OutDataTypeStr=boolean
  Long_Accel_Val : Outport  VectorParamsAs1DForOutWhenUnconnected=off
  wires:
  Logical Operator1/1 -> Logical Operator5/1
  Label205_Corrupted/1 -> Logical Operator1/3
  Label205_SSM/1 -> Compare To Constant/1
  Label205_Not_Refreshed/1 -> Logical Operator1/2
  DFCSB_Long_Accel/1 -> Compare To Constant4/1, Compare To Constant3/1
  Compare To Constant3/1 -> Logical Operator1/5
  Capsule_Validity/1 -> Compare To Zero/1
  Compare To Zero/1 -> Logical Operator1/1
  Compare To Constant/1 -> Logical Operator1/4
  Compare To Constant4/1 -> Logical Operator1/6
  Logical Operator5/1 -> Long_Accel_Val/1

== system MATLAB_TEST/AVIONICS/Brake_Control_Module_Side_A/BCSA Controller CP/DFCS3_Label206_Validity ==
  Capsule_Validity : Inport
  Label206_Not_Refreshed : Inport  Port=2
  Label206_Corrupted : Inport  Port=3
  Label206_SSM : Inport  Port=4
  DFCSB_Gnd_Spd : Inport  Port=5
  Compare To Constant : simulink/Logic and Bit Operations/Compare To Constant  relop=~=  const=3.0  OutDataTypeStr=boolean
  Compare To Constant3 : simulink/Logic and Bit Operations/Compare To Constant  relop=<  const=0  OutDataTypeStr=boolean
  Compare To Constant4 : simulink/Logic and Bit Operations/Compare To Constant  relop=>  const=4096  OutDataTypeStr=boolean
  Compare To Zero : simulink/Logic and Bit Operations/Compare To Zero  relop===  OutDataTypeStr=boolean
  Logical Operator : Logic  Operator=OR  Inputs=6  AllPortsSameDT=off  OutDataTypeStr=boolean
  Logical Operator5 : Logic  Operator=NOT  AllPortsSameDT=off  OutDataTypeStr=boolean
  Gnd_Spd_Val : Outport  VectorParamsAs1DForOutWhenUnconnected=off
  wires:
  Compare To Constant3/1 -> Logical Operator/5
  DFCSB_Gnd_Spd/1 -> Compare To Constant4/1, Compare To Constant3/1
  Compare To Zero/1 -> Logical Operator/1
  Logical Operator/1 -> Logical Operator5/1
  Label206_Corrupted/1 -> Logical Operator/3
  Label206_Not_Refreshed/1 -> Logical Operator/2
  Capsule_Validity/1 -> Compare To Zero/1
  Label206_SSM/1 -> Compare To Constant/1
  Compare To Constant4/1 -> Logical Operator/6
  Compare To Constant/1 -> Logical Operator/4
  Logical Operator5/1 -> Gnd_Spd_Val/1

== system MATLAB_TEST/AVIONICS/Brake_Control_Module_Side_A/BCSA Controller CP/DFCS3_Label207_Validity ==
  Capsule_Validity : Inport
  Label207_Not_Refreshed : Inport  Port=2
  Label207_Corrupted : Inport  Port=3
  Label207_SSM : Inport  Port=4
  DFCSB_Pitch_Ang : Inport  Port=5
  Compare To Constant : simulink/Logic and Bit Operations/Compare To Constant  relop=~=  const=3.0  OutDataTypeStr=boolean
  Compare To Constant3 : simulink/Logic and Bit Operations/Compare To Constant  relop=<  const=-90  OutDataTypeStr=boolean
  Compare To Constant4 : simulink/Logic and Bit Operations/Compare To Constant  relop=>  const=90  OutDataTypeStr=boolean
  Compare To Zero : simulink/Logic and Bit Operations/Compare To Zero  relop===  OutDataTypeStr=boolean
  Logical Operator1 : Logic  Operator=OR  Inputs=6  AllPortsSameDT=off  OutDataTypeStr=boolean
  Logical Operator5 : Logic  Operator=NOT  AllPortsSameDT=off  OutDataTypeStr=boolean
  Pitch_Ang_Val : Outport  VectorParamsAs1DForOutWhenUnconnected=off
  wires:
  Compare To Zero/1 -> Logical Operator1/1
  Compare To Constant/1 -> Logical Operator1/4
  Label207_SSM/1 -> Compare To Constant/1
  Label207_Corrupted/1 -> Logical Operator1/3
  Compare To Constant3/1 -> Logical Operator1/5
  Compare To Constant4/1 -> Logical Operator1/6
  DFCSB_Pitch_Ang/1 -> Compare To Constant4/1, Compare To Constant3/1
  Capsule_Validity/1 -> Compare To Zero/1
  Label207_Not_Refreshed/1 -> Logical Operator1/2
  Logical Operator1/1 -> Logical Operator5/1
  Logical Operator5/1 -> Pitch_Ang_Val/1

== system MATLAB_TEST/AVIONICS/Brake_Control_Module_Side_A/BCSA Controller CP/DFCSA_DCL_Inhibition_Comp ==
  DCL_Inhibition : Inport
  DCL_Inhibition_Val : Inport  Port=2
  Compare To Zero : simulink/Logic and Bit Operations/Compare To Zero  relop===  OutDataTypeStr=boolean
  Init: 0 : UnitDelay  SampleTime=-1  HasFrameUpgradeWarning=on
  Switch : Switch  Criteria=u2 > Threshold
  DCL_Inhibition_out : Outport  VectorParamsAs1DForOutWhenUnconnected=off
  wires:
  Init: 0/1 -> Switch/1
  Switch/1 -> DCL_Inhibition_out/1, Init: 0/1
  DCL_Inhibition/1 -> Switch/3
  Compare To Zero/1 -> Switch/2
  DCL_Inhibition_Val/1 -> Compare To Zero/1

== system MATLAB_TEST/AVIONICS/Brake_Control_Module_Side_A/BCSA Controller CP/DFCSA_Ground_Speed_Comp ==
  Ground_Speed : Inport
  Ground_Speed_Val : Inport  Port=2
  Compare To Zero : simulink/Logic and Bit Operations/Compare To Zero  relop===  OutDataTypeStr=boolean
  Init: 0 : UnitDelay  SampleTime=-1  HasFrameUpgradeWarning=on
  Switch : Switch  Criteria=u2 > Threshold
  Ground_Speed_out : Outport  VectorParamsAs1DForOutWhenUnconnected=off
  wires:
  Init: 0/1 -> Switch/1
  Switch/1 -> Ground_Speed_out/1, Init: 0/1
  Ground_Speed/1 -> Switch/3
  Compare To Zero/1 -> Switch/2
  Ground_Speed_Val/1 -> Compare To Zero/1

== system MATLAB_TEST/AVIONICS/Brake_Control_Module_Side_A/BCSA Controller CP/DFCSA_LH_Braking_Cmd_Comp ==
  Braking_Cmd : Inport
  Braking_Cmd_Val : Inport  Port=2
  Compare To Zero : simulink/Logic and Bit Operations/Compare To Zero  relop===  OutDataTypeStr=boolean
  Init: 0 : UnitDelay  SampleTime=-1  HasFrameUpgradeWarning=on
  Switch : Switch  Criteria=u2 > Threshold
  Braking_Cmd_out : Outport  VectorParamsAs1DForOutWhenUnconnected=off
  wires:
  Braking_Cmd_Val/1 -> Compare To Zero/1
  Compare To Zero/1 -> Switch/2
  Braking_Cmd/1 -> Switch/3
  Switch/1 -> Init: 0/1, Braking_Cmd_out/1
  Init: 0/1 -> Switch/1

== system MATLAB_TEST/AVIONICS/Brake_Control_Module_Side_A/BCSA Controller CP/DFCSA_LMLG_WOWs_Comp ==
  LMLG_WOWs : Inport
  LMLG_WOWs_Val : Inport  Port=2
  Compare To Zero : simulink/Logic and Bit Operations/Compare To Zero  relop===  OutDataTypeStr=boolean
  Init: 0 : UnitDelay  SampleTime=-1  HasFrameUpgradeWarning=on
  Switch : Switch  Criteria=u2 > Threshold
  LMLG_WOWs_out : Outport  VectorParamsAs1DForOutWhenUnconnected=off
  wires:
  Init: 0/1 -> Switch/1
  Switch/1 -> LMLG_WOWs_out/1, Init: 0/1
  LMLG_WOWs/1 -> Switch/3
  Compare To Zero/1 -> Switch/2
  LMLG_WOWs_Val/1 -> Compare To Zero/1

== system MATLAB_TEST/AVIONICS/Brake_Control_Module_Side_A/BCSA Controller CP/DFCSA_Label202_Validity ==
  Capsule_Validity : Inport
  Label202_Not_Refreshed : Inport  Port=2
  Label202_Corrupted : Inport  Port=3
  Label202_SSM : Inport  Port=4
  DFCSA_LH_Braking_Cmd : Inport  Port=5
  DFCSA_RH_Braking_Cmd : Inport  Port=6
  Compare To Constant : simulink/Logic and Bit Operations/Compare To Constant  relop=~=  const=3.0  OutDataTypeStr=boolean
  Compare To Constant1 : simulink/Logic and Bit Operations/Compare To Constant  relop=<  const=0  OutDataTypeStr=boolean
  Compare To Constant2 : simulink/Logic and Bit Operations/Compare To Constant  relop=>  const=100  OutDataTypeStr=boolean
  Compare To Constant3 : simulink/Logic and Bit Operations/Compare To Constant  relop=<  const=0  OutDataTypeStr=boolean
  Compare To Constant4 : simulink/Logic and Bit Operations/Compare To Constant  relop=>  const=100  OutDataTypeStr=boolean
  Compare To Zero : simulink/Logic and Bit Operations/Compare To Zero  relop===  OutDataTypeStr=boolean
  Logical Operator : Logic  Operator=OR  Inputs=4  AllPortsSameDT=off  OutDataTypeStr=boolean
  Logical Operator{1..4} (4 alike) : Logic  Operator=OR  AllPortsSameDT=off  OutDataTypeStr=boolean
  Logical Operator5 : Logic  Operator=NOT  AllPortsSameDT=off  OutDataTypeStr=boolean
  Logical Operator6 : Logic  Operator=NOT  AllPortsSameDT=off  OutDataTypeStr=boolean
  LH_Braking_Cmd_Val : Outport  VectorParamsAs1DForOutWhenUnconnected=off
  RH_Braking_Cmd_Val : Outport  Port=2  VectorParamsAs1DForOutWhenUnconnected=off
  wires:
  Label202_Not_Refreshed/1 -> Logical Operator/2
  Compare To Zero/1 -> Logical Operator/1
  Capsule_Validity/1 -> Compare To Zero/1
  Label202_Corrupted/1 -> Logical Operator/3
  Label202_SSM/1 -> Compare To Constant/1
  Compare To Constant/1 -> Logical Operator/4
  Logical Operator/1 -> Logical Operator4/1, Logical Operator2/2
  DFCSA_LH_Braking_Cmd/1 -> Compare To Constant2/1, Compare To Constant1/1
  Compare To Constant2/1 -> Logical Operator1/1
  Compare To Constant1/1 -> Logical Operator1/2
  Logical Operator1/1 -> Logical Operator2/1
  Logical Operator2/1 -> Logical Operator5/1
  Compare To Constant3/1 -> Logical Operator3/2
  Compare To Constant4/1 -> Logical Operator3/1
  DFCSA_RH_Braking_Cmd/1 -> Compare To Constant3/1, Compare To Constant4/1
  Logical Operator3/1 -> Logical Operator4/2
  Logical Operator4/1 -> Logical Operator6/1
  Logical Operator5/1 -> LH_Braking_Cmd_Val/1
  Logical Operator6/1 -> RH_Braking_Cmd_Val/1

== system MATLAB_TEST/AVIONICS/Brake_Control_Module_Side_A/BCSA Controller CP/DFCSA_Long_Accel_Comp ==
  Long_Accel : Inport
  Long_Accel_Val : Inport  Port=2
  Compare To Zero : simulink/Logic and Bit Operations/Compare To Zero  relop===  OutDataTypeStr=boolean
  Init: -0.61 : UnitDelay  InitialCondition=double(single(-0.61))  SampleTime=-1  HasFrameUpgradeWarning=on
  Switch : Switch  Criteria=u2 > Threshold
  Long_Accel_out : Outport  VectorParamsAs1DForOutWhenUnconnected=off
  wires:
  Long_Accel_Val/1 -> Compare To Zero/1
  Compare To Zero/1 -> Switch/2
  Long_Accel/1 -> Switch/3
  Switch/1 -> Init: -0.61/1, Long_Accel_out/1
  Init: -0.61/1 -> Switch/1

== system MATLAB_TEST/AVIONICS/Brake_Control_Module_Side_A/BCSA Controller CP/DFCSA_NLG_WOWs_Comp ==
  NLG_WOWs : Inport
  NLG_WOWs_Val : Inport  Port=2
  Compare To Zero : simulink/Logic and Bit Operations/Compare To Zero  relop===  OutDataTypeStr=boolean
  Init: 0 : UnitDelay  SampleTime=-1  HasFrameUpgradeWarning=on
  Switch : Switch  Criteria=u2 > Threshold
  NLG_WOWs_out : Outport  VectorParamsAs1DForOutWhenUnconnected=off
  wires:
  NLG_WOWs_Val/1 -> Compare To Zero/1
  Compare To Zero/1 -> Switch/2
  NLG_WOWs/1 -> Switch/3
  Switch/1 -> Init: 0/1, NLG_WOWs_out/1
  Init: 0/1 -> Switch/1

== system MATLAB_TEST/AVIONICS/Brake_Control_Module_Side_A/BCSA Controller CP/DFCSA_Pitch_Angle_Comp ==
  Pitch_Angle : Inport
  Pitch_Angle_Val : Inport  Port=2
  Compare To Zero : simulink/Logic and Bit Operations/Compare To Zero  relop===  OutDataTypeStr=boolean
  Init: 0 : UnitDelay  SampleTime=-1  HasFrameUpgradeWarning=on
  Switch : Switch  Criteria=u2 > Threshold
  Pitch_Angle_out : Outport  VectorParamsAs1DForOutWhenUnconnected=off
  wires:
  Init: 0/1 -> Switch/1
  Switch/1 -> Pitch_Angle_out/1, Init: 0/1
  Pitch_Angle/1 -> Switch/3
  Compare To Zero/1 -> Switch/2
  Pitch_Angle_Val/1 -> Compare To Zero/1

== system MATLAB_TEST/AVIONICS/Brake_Control_Module_Side_A/BCSA Controller CP/DFCSA_RH_Braking_Cmd_Comp ==
  Braking_Cmd : Inport
  Braking_Cmd_Val : Inport  Port=2
  Compare To Zero : simulink/Logic and Bit Operations/Compare To Zero  relop===  OutDataTypeStr=boolean
  Init: 0 : UnitDelay  SampleTime=-1  HasFrameUpgradeWarning=on
  Switch : Switch  Criteria=u2 > Threshold
  Braking_Cmd_out : Outport  VectorParamsAs1DForOutWhenUnconnected=off
  wires:
  Init: 0/1 -> Switch/1
  Switch/1 -> Braking_Cmd_out/1, Init: 0/1
  Braking_Cmd/1 -> Switch/3
  Compare To Zero/1 -> Switch/2
  Braking_Cmd_Val/1 -> Compare To Zero/1

== system MATLAB_TEST/AVIONICS/Brake_Control_Module_Side_A/BCSA Controller CP/DFCSA_RMLG_WOWs_Comp ==
  RMLG_WOWs : Inport
  RMLG_WOWs_Val : Inport  Port=2
  Compare To Zero : simulink/Logic and Bit Operations/Compare To Zero  relop===  OutDataTypeStr=boolean
  Init: 0 : UnitDelay  SampleTime=-1  HasFrameUpgradeWarning=on
  Switch : Switch  Criteria=u2 > Threshold
  RMLG_WOWs_out : Outport  VectorParamsAs1DForOutWhenUnconnected=off
  wires:
  Init: 0/1 -> Switch/1
  Switch/1 -> RMLG_WOWs_out/1, Init: 0/1
  RMLG_WOWs/1 -> Switch/3
  Compare To Zero/1 -> Switch/2
  RMLG_WOWs_Val/1 -> Compare To Zero/1

== system MATLAB_TEST/AVIONICS/Brake_Control_Module_Side_A/BCSA Controller CP/DFCSA_TLA_Above_Idle_Comp ==
  TLA_Above_Idle : Inport
  TLA_Above_Idle_Val : Inport  Port=2
  Compare To Zero : simulink/Logic and Bit Operations/Compare To Zero  relop===  OutDataTypeStr=boolean
  Init: 0 : UnitDelay  SampleTime=-1  HasFrameUpgradeWarning=on
  Switch : Switch  Criteria=u2 > Threshold
  TLA_Above_Idle_out : Outport  VectorParamsAs1DForOutWhenUnconnected=off
  wires:
  TLA_Above_Idle_Val/1 -> Compare To Zero/1
  Compare To Zero/1 -> Switch/2
  TLA_Above_Idle/1 -> Switch/3
  Switch/1 -> Init: 0/1, TLA_Above_Idle_out/1
  Init: 0/1 -> Switch/1

== system MATLAB_TEST/AVIONICS/Brake_Control_Module_Side_A/BCSA Controller CP/DFCSA_WOWs_Val_Comp ==
  WOWs_Val_Acq : Inport
  WOWs_Val_Val : Inport  Port=2
  Compare To Zero : simulink/Logic and Bit Operations/Compare To Zero  relop===  OutDataTypeStr=boolean
  Init: 0 : UnitDelay  SampleTime=-1  HasFrameUpgradeWarning=on
  Switch : Switch  Criteria=u2 > Threshold
  WOWs_Val_Acq_out : Outport  VectorParamsAs1DForOutWhenUnconnected=off
  wires:
  WOWs_Val_Val/1 -> Compare To Zero/1
  Compare To Zero/1 -> Switch/2
  WOWs_Val_Acq/1 -> Switch/3
  Switch/1 -> Init: 0/1, WOWs_Val_Acq_out/1
  Init: 0/1 -> Switch/1

== system MATLAB_TEST/AVIONICS/Brake_Control_Module_Side_A/BCSA Controller CP/DFCSB_DCL_Inhibition_Comp ==
  DCL_Inhibition : Inport
  DCL_Inhibition_Val : Inport  Port=2
  Compare To Zero : simulink/Logic and Bit Operations/Compare To Zero  relop===  OutDataTypeStr=boolean
  Init: 0 : UnitDelay  SampleTime=-1  HasFrameUpgradeWarning=on
  Switch : Switch  Criteria=u2 > Threshold
  DCL_Inhibition_out : Outport  VectorParamsAs1DForOutWhenUnconnected=off
  wires:
  DCL_Inhibition_Val/1 -> Compare To Zero/1
  Compare To Zero/1 -> Switch/2
  DCL_Inhibition/1 -> Switch/3
  Switch/1 -> Init: 0/1, DCL_Inhibition_out/1
  Init: 0/1 -> Switch/1

== system MATLAB_TEST/AVIONICS/Brake_Control_Module_Side_A/BCSA Controller CP/DFCSB_Ground_Speed_Comp ==
  Ground_Speed : Inport
  Ground_Speed_Val : Inport  Port=2
  Compare To Zero : simulink/Logic and Bit Operations/Compare To Zero  relop===  OutDataTypeStr=boolean
  Init: 0 : UnitDelay  SampleTime=-1  HasFrameUpgradeWarning=on
  Switch : Switch  Criteria=u2 > Threshold
  Ground_Speed_out : Outport  VectorParamsAs1DForOutWhenUnconnected=off
  wires:
  Ground_Speed_Val/1 -> Compare To Zero/1
  Compare To Zero/1 -> Switch/2
  Ground_Speed/1 -> Switch/3
  Switch/1 -> Init: 0/1, Ground_Speed_out/1
  Init: 0/1 -> Switch/1

== system MATLAB_TEST/AVIONICS/Brake_Control_Module_Side_A/BCSA Controller CP/DFCSB_LH_Braking_Cmd_Comp ==
  Braking_Cmd : Inport
  Braking_Cmd_Val : Inport  Port=2
  Compare To Zero : simulink/Logic and Bit Operations/Compare To Zero  relop===  OutDataTypeStr=boolean
  Init: 0 : UnitDelay  SampleTime=-1  HasFrameUpgradeWarning=on
  Switch : Switch  Criteria=u2 > Threshold
  Braking_Cmd_out : Outport  VectorParamsAs1DForOutWhenUnconnected=off
  wires:
  Init: 0/1 -> Switch/1
  Switch/1 -> Braking_Cmd_out/1, Init: 0/1
  Braking_Cmd/1 -> Switch/3
  Compare To Zero/1 -> Switch/2
  Braking_Cmd_Val/1 -> Compare To Zero/1

== system MATLAB_TEST/AVIONICS/Brake_Control_Module_Side_A/BCSA Controller CP/DFCSB_LMLG_WOWs_Comp ==
  LMLG_WOWs : Inport
  LMLG_WOWs_Val : Inport  Port=2
  Compare To Zero : simulink/Logic and Bit Operations/Compare To Zero  relop===  OutDataTypeStr=boolean
  Init: 0 : UnitDelay  SampleTime=-1  HasFrameUpgradeWarning=on
  Switch : Switch  Criteria=u2 > Threshold
  LMLG_WOWs_out : Outport  VectorParamsAs1DForOutWhenUnconnected=off
  wires:
  LMLG_WOWs_Val/1 -> Compare To Zero/1
  Compare To Zero/1 -> Switch/2
  LMLG_WOWs/1 -> Switch/3
  Switch/1 -> Init: 0/1, LMLG_WOWs_out/1
  Init: 0/1 -> Switch/1
